simulink model "qddot"  (R2018b)
settings: Solver=ode5  StartTime=0.0  StopTime=10.0  FixedStep=0.001  RelTol=1e-3
settings Model: Creator=tfu3  LastModifiedBy=Tianshi_Fu
settings DebuggingCC: LibraryContextMissingDiagnostic=none
settings SFSimCC: SimUseLocalCustomCode=off
settings RTWCC: RTWUseLocalCustomCode=off

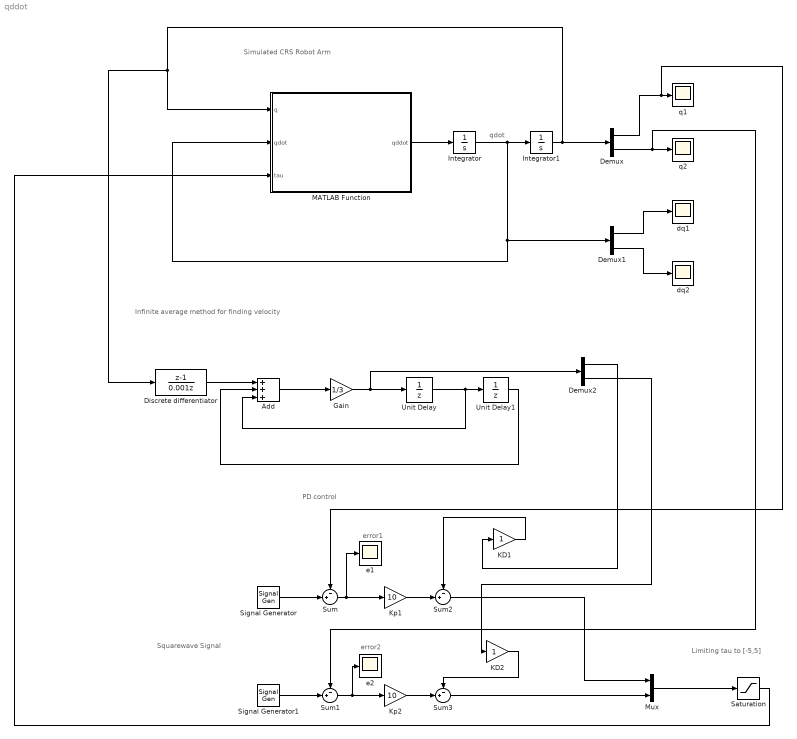
== system qddot ==
  note: Limiting tau to [-5,5]
  note: error2
  note: error1
  note: qdot
  note: Simulated CRS Robot Arm
  note: PD control
  note: Infinite average method for finding velocity
  note: Squarewave Signal
  Add : Sum  Inputs=+++
  Demux : Demux  Outputs=2
  Demux1 : Demux  Outputs=2
  Demux2 : Demux  Outputs=2
  Discrete differentiator : DiscreteTransferFcn  Numerator=[1 -1]  Denominator=[0.001 0]  SampleTime=0.001
  Gain : Gain  Gain=1/3
  Integrator : Integrator  InitialCondition=[0;0]
  Integrator1 : Integrator  InitialCondition=[pi/2;0]
  KD1 : Gain
  KD2 : Gain
  Kp1 : Gain  Gain=10
  Kp2 : Gain  Gain=10
  MATLAB Function : MATLAB Function  TreatAsAtomicUnit=on
  Mux : Mux  Inputs=2
  Saturation : Saturate  UpperLimit=5  LowerLimit=-5
  Signal Generator : SignalGenerator  WaveForm=square  Amplitude=pi/6  Frequency=0.5
  Signal Generator1 : SignalGenerator  WaveForm=square  Amplitude=pi/6  Frequency=0.5
  Sum{,1..3} (4 alike) : Sum  Inputs=-+|
  Unit Delay : UnitDelay  SampleTime=0.001
  Unit Delay1 : UnitDelay  SampleTime=0.001
  dq1 : Scope
  dq2 : Scope
  e1 : Scope
  e2 : Scope
  q1 : Scope
  q2 : Scope
  wires:
  MATLAB Function/1(qddot) -> Integrator/1
  Integrator/1 -> Demux1/1, MATLAB Function/2(qdot), Integrator1/1
  Integrator1/1 -> Demux/1, Discrete differentiator/1, MATLAB Function/1(q)
  Demux/1 -> Sum/1, q1/1
  Demux1/1 -> dq1/1
  Demux1/2 -> dq2/1
  Discrete differentiator/1 -> Add/1
  Unit Delay/1 -> Add/3, Unit Delay1/1
  Unit Delay1/1 -> Add/2
  Gain/1 -> Demux2/1, Unit Delay/1
  Add/1 -> Gain/1
  Signal Generator/1 -> Sum/2
  Sum/1 -> e1/1, Kp1/1
  Signal Generator1/1 -> Sum1/2
  Demux/2 -> Sum1/1, q2/1
  Kp1/1 -> Sum2/2
  Kp2/1 -> Sum3/2
  KD1/1 -> Sum2/1
  KD2/1 -> Sum3/1
  Sum2/1 -> Mux/1
  Sum3/1 -> Mux/2
  Mux/1 -> Saturation/1
  Saturation/1 -> MATLAB Function/3(tau)
  Sum1/1 -> e2/1, Kp2/1
  Demux2/1 -> KD1/1
  Demux2/2 -> KD2/1

== matlab function qddot/MATLAB Function ==
  data: q input; qddot output; qdot input; tau input
function qddot = fcn(q,qdot,tau)

p = [0.0300; 0.0128; 0.0076; 0.0753; 0.0298];
g = 9.805;


D = [p(1) -p(3)*sin(q(2)-q(1)); -p(3)*sin(q(2)-q(1)) p(2)];
C = [0 -p(3)*cos(q(2)-q(1))*qdot(2); p(3)*cos(q(2)-q(1))*qdot(1) 0];
G = [-p(4)*g*sin(q(1)); -p(5)*g*cos(q(2))];

qddot = inv(D)*tau - inv(D)*C*qdot - inv(D)*G;
